simulink model "STFT_IP"  (R2021b)
settings: Solver=VariableStepAuto  StartTime=0.0  StopTime=2048*15/fs  RelTol=1e-3
InitFcn:
  | f = 12.288e6;
  | fs = 61.44e6;
  | N = 8;
  | n = 0:N-1;
  | Hamming = 0.54 - 0.46 * cos(2*pi*n/N);
  | Norm_Ham = sum(Hamming);
  | Hanning = 0.5 * (1 + cos(2*pi*n/N));
  | Norm_Han = sum(Hanning);
libraries: hdlBasic x52, hdlDSPIP x1, hdlsllib x1, vmcUtilities x1
settings Model: Creator=yxb20126  LastModifiedBy=yxb20126

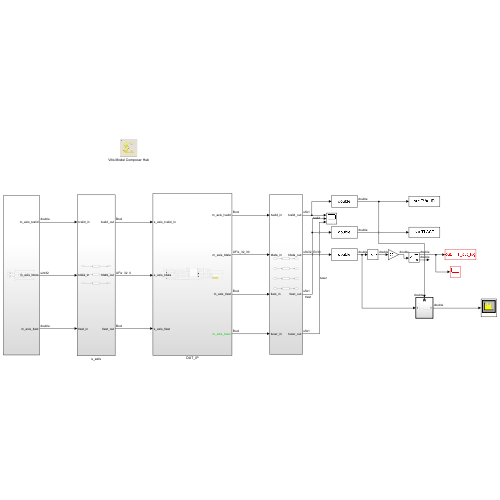
[thumbnail: Simulink's stored preview of the top-level diagram]
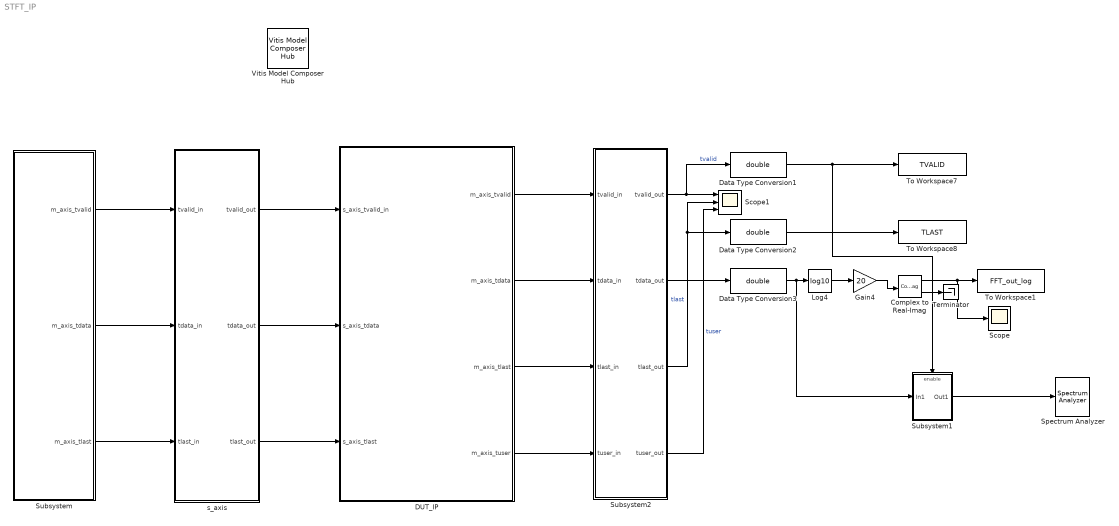
== system STFT_IP ==
  Complex to Real-Imag : ComplexToRealImag
  DUT_IP : Subsystem
  Data Type Conversion1 : DataTypeConversion  OutDataTypeStr=double  SaturateOnIntegerOverflow=on
  Data Type Conversion2 : DataTypeConversion  OutDataTypeStr=double  SaturateOnIntegerOverflow=on
  Data Type Conversion3 : DataTypeConversion  OutDataTypeStr=double  SaturateOnIntegerOverflow=on
  Gain4 : Gain  Gain=20
  Log4 : Math  Operator=log10  OutputSignalType=real  SaturateOnIntegerOverflow=on
  Scope : Scope
  Scope1 : Scope  NumInputPorts=3
  Spectrum Analyzer : SpectrumAnalyzer  IsFrequencyInputMode=1
  Subsystem : Subsystem
  Subsystem1 : Subsystem
  Subsystem2 : Subsystem
  Terminator : Terminator
  To Workspace1 : ToWorkspace  VariableName=FFT_out_log  SampleTime=-1
      settings: Save2DSignal=2-D array (concatenate along first dimension)
  To Workspace7 : ToWorkspace  VariableName=TVALID  SampleTime=1/fs
      settings: Save2DSignal=2-D array (concatenate along first dimension)
  To Workspace8 : ToWorkspace  VariableName=TLAST  SampleTime=1/fs
      settings: Save2DSignal=2-D array (concatenate along first dimension)
  Vitis Model Composer Hub : vmcUtilities/Vitis Model Composer Hub  Tag=genX  CodeGeneration=off  SubsystemName=<enter or select subsystem name>  TargetDirectory=./code  ExportType=HLS C++ code  IpVendor=xilinx.com  IpLibrary=hls  IpVersion=1.0  IpHWLanguage=Verilog  AieCompilerOptions={}  CreateTestbench=off  TestbenchStackSize=10  RunAieSim=off  AieSimTimeout=50000  RunAieSimProfiling=off  LaunchVitisAnalyzer=off  PlotOutput=off  RunX86Sim=off  X86SimTimeout=10  GenHwImage=off  PlatformType=Not Specified  HwSystemType=Baremetal  HwValidationTarget=hw  ProjDevice=xczu48dr-ffvg1517-2-e  ProjDevicePart=xczu48dr-ffvg1517-2-e  SamplePeriod=-1  ClockFrequency=200  DataPathParallelism=1  xilinxfamily=zynquplusRFSOC  part=xczu48dr  speed=-2-e  package=ffvg1517  directory=C:/Workspace/STFT  testbench=off  incr_netlist=off  synthesis_tool=Vivado  clock_wrapper=Clock Enables  dbl_ovrd=According to Block Masks  dcm_input_clock_period=10  sysclk_period=(1/fs)*10e9  simulink_period=1/fs  eval_field=0
  s_axis : Subsystem
  wires:
  Subsystem/1(m_axis_tvalid) -> s_axis/1(tvalid_in)
  Subsystem/2(m_axis_tdata) -> s_axis/2(tdata_in)
  Subsystem/3(m_axis_tlast) -> s_axis/3(tlast_in)
  s_axis/1(tvalid_out) -> DUT_IP/1(s_axis_tvalid_in)
  s_axis/2(tdata_out) -> DUT_IP/2(s_axis_tdata)
  s_axis/3(tlast_out) -> DUT_IP/3(s_axis_tlast)
  DUT_IP/4(m_axis_tuser) -> Subsystem2/4(tuser_in)
  Subsystem2/2(tdata_out) -> Data Type Conversion3/1
  Subsystem2/1(tvalid_out) -> Data Type Conversion1/1, Scope1/1  "tvalid"
  Subsystem2/3(tlast_out) -> Scope1/2, Data Type Conversion2/1  "tlast"
  Subsystem2/4(tuser_out) -> Scope1/3  "tuser"
  Data Type Conversion1/1 -> Subsystem1/Enable, To Workspace7/1
  Data Type Conversion2/1 -> To Workspace8/1
  Log4/1 -> Gain4/1
  Data Type Conversion3/1 -> Subsystem1/1(In1), Log4/1
  DUT_IP/1(m_axis_tvalid) -> Subsystem2/1(tvalid_in)
  DUT_IP/2(m_axis_tdata) -> Subsystem2/2(tdata_in)
  DUT_IP/3(m_axis_tlast) -> Subsystem2/3(tlast_in)
  Gain4/1 -> Complex to Real-Imag/1
  Complex to Real-Imag/1 -> Scope/1, To Workspace1/1
  Complex to Real-Imag/2 -> Terminator/1
  Subsystem1/1(Out1) -> Spectrum Analyzer/1

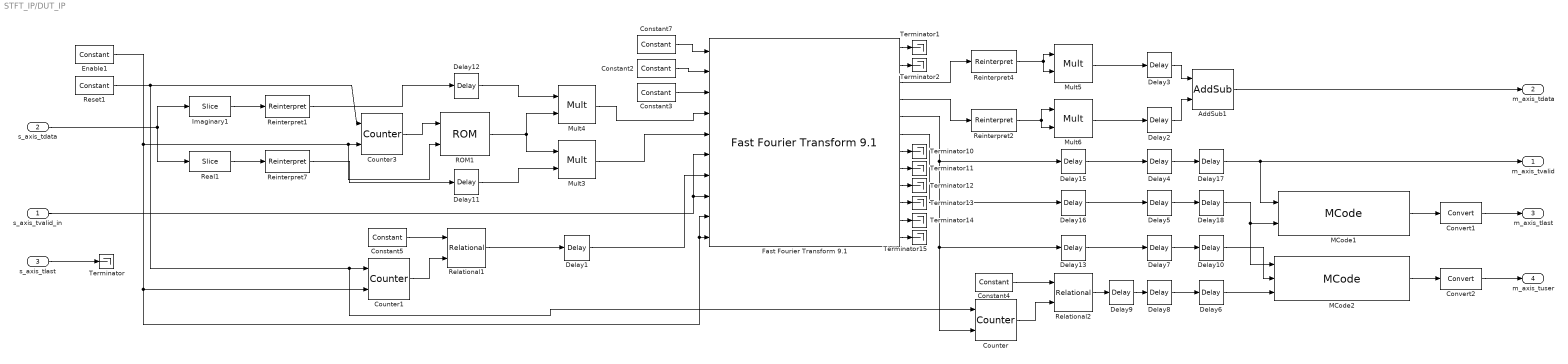
== system STFT_IP/DUT_IP ==
  s_axis_tvalid_in : Inport
  s_axis_tdata : Inport  Port=2
  s_axis_tlast : Inport  Port=3
  AddSub1 : hdlBasic/AddSub  mode=Addition  use_carryin=off  use_carryout=off  en=off  latency=1  precision=User Defined  arith_type=Unsigned  n_bits=32  bin_pt=30  quantization=Truncate  overflow=Saturate  use_behavioral_HDL=off  hw_selection=Fabric  pipelined=off  XmcBlockStatus=1  maskContainerNames=tabcontainer1  block_type=addsub  block_config=sysgen:Addsub_config
  Constant2 : hdlBasic/Constant  const=0  gui_display_data_type=Fixed-point  arith_type=Unsigned  n_bits=1  bin_pt=0  preci_type=Single  exp_width=8  frac_width=24  explicit_period=on  period=1/fs  XmcBlockStatus=1  maskContainerNames=tabcontainer1  block_type=constant  block_config=sysgen:Constant_config
  Constant3 : hdlBasic/Constant  const=0  gui_display_data_type=Boolean  arith_type=Boolean  n_bits=1  bin_pt=0  preci_type=Single  exp_width=8  frac_width=24  explicit_period=on  period=1/fs  XmcBlockStatus=1  maskContainerNames=tabcontainer1  block_type=constant  block_config=sysgen:Constant_config
  Constant4 : hdlBasic/Constant  const=N*1024-1  gui_display_data_type=Fixed-point  arith_type=Unsigned  n_bits=ceil(log2(N*1024))  bin_pt=0  preci_type=Single  exp_width=8  frac_width=24  explicit_period=on  period=1/fs  XmcBlockStatus=1  maskContainerNames=tabcontainer1  block_type=constant  block_config=sysgen:Constant_config
  Constant5 : hdlBasic/Constant  const=N-1  gui_display_data_type=Fixed-point  arith_type=Unsigned  n_bits=11  bin_pt=0  preci_type=Single  exp_width=8  frac_width=24  explicit_period=on  period=1/fs  XmcBlockStatus=1  maskContainerNames=tabcontainer1  block_type=constant  block_config=sysgen:Constant_config
  Constant7 : hdlBasic/Constant  const=0  gui_display_data_type=Fixed-point  arith_type=Unsigned  n_bits=12  bin_pt=0  preci_type=Single  exp_width=8  frac_width=24  explicit_period=on  period=1/fs  XmcBlockStatus=1  maskContainerNames=tabcontainer1  block_type=constant  block_config=sysgen:Constant_config
  Convert1 : hdlBasic/Convert  gui_display_data_type=Boolean  arith_type=Boolean  n_bits=16  bin_pt=14  float_type=Single  exp_bits=8  fraction_bits=24  quantization=Truncate  overflow=Wrap  en=off  latency=0  pipeline=off  XmcBlockStatus=1  maskContainerNames=group2  block_type=convert  block_config=sysgen:Convert_config
  Convert2 : hdlBasic/Convert  gui_display_data_type=Boolean  arith_type=Boolean  n_bits=16  bin_pt=14  float_type=Single  exp_bits=8  fraction_bits=24  quantization=Truncate  overflow=Wrap  en=off  latency=0  pipeline=off  XmcBlockStatus=1  maskContainerNames=group2  block_type=convert  block_config=sysgen:Convert_config
  Counter : hdlBasic/Counter  cnt_type=Count limited  cnt_to=N*1024-1  operation=Up  start_count=0  cnt_by_val=1  arith_type=Unsigned  n_bits=ceil(log2(N*1024))  bin_pt=0  load_pin=off  rst=on  en=on  explicit_period=Explicit  period=1/fs  use_behavioral_HDL=off  implementation=Fabric  XmcBlockStatus=1  maskContainerNames=group1  block_type=counter  block_config=sysgen:Counter_config
  Counter1 : hdlBasic/Counter  cnt_type=Count limited  cnt_to=N-1  operation=Up  start_count=0  cnt_by_val=1  arith_type=Unsigned  n_bits=11  bin_pt=0  load_pin=off  rst=on  en=on  explicit_period=Explicit  period=1/fs  use_behavioral_HDL=off  implementation=Fabric  XmcBlockStatus=1  maskContainerNames=group1  block_type=counter  block_config=sysgen:Counter_config
  Counter3 : hdlBasic/Counter  cnt_type=Count limited  cnt_to=N-1  operation=Up  start_count=0  cnt_by_val=1  arith_type=Unsigned  n_bits=ceil(log2(N))  bin_pt=0  load_pin=off  rst=on  en=on  explicit_period=Explicit  period=1/fs  use_behavioral_HDL=off  implementation=Fabric  XmcBlockStatus=1  maskContainerNames=group1  block_type=counter  block_config=sysgen:Counter_config
  Delay{1,13,15..16} (4 alike) : hdlBasic/Delay  rst=off  en=off  latency=3  reg_retiming=off  XmcBlockStatus=1  maskContainerNames=group1  block_type=delay  block_config=sysgen:Delay_config
  Delay{2..8,10..12,17..18} (12 alike) : hdlBasic/Delay  rst=off  en=off  latency=1  reg_retiming=off  XmcBlockStatus=1  maskContainerNames=group1  block_type=delay  block_config=sysgen:Delay_config
  Delay9 : hdlBasic/Delay  rst=off  en=off  latency=2  reg_retiming=off  XmcBlockStatus=1  maskContainerNames=group1  block_type=delay  block_config=sysgen:Delay_config
  Enable1 : hdlBasic/Constant  const=1  gui_display_data_type=Boolean  arith_type=Boolean  n_bits=11  bin_pt=0  preci_type=Single  exp_width=8  frac_width=24  explicit_period=on  period=1/fs  XmcBlockStatus=1  maskContainerNames=tabcontainer1  block_type=constant  block_config=sysgen:Constant_config
  Fast Fourier Transform 9.1 : hdlDSPIP/Fast Fourier Transform 9.1   transform_length=2048  target_clock_frequency=200  target_data_throughput=50  implementation_options=pipelined_streaming_io  run_time_configurable_transform_length=off  phase_factor_width=16  scaling_options=scaled  rounding_modes=truncation  aclken=on  aresetn=on  output_ordering=natural_order  cyclic_prefix_insertion=off  throttle_scheme=nonrealtime  xk_index=off  ovflo=off  trim_axipin_name=on  memory_options_data=block_ram  memory_options_phase_factors=block_ram  number_of_stages_using_block_ram_for_data_and_phase_factors=6  memory_options_reorder=block_ram  memory_options_hybrid=off  complex_mult_type=use_mults_resources  butterfly_type=use_luts  simulation_type=hybrid_sim  simulation_model=sysgen:xfftv9_cmodel  data_path_portlist={ 's_axis_data_tdata', 'm_axis_data_tdata', 'm_axis_status_tdata', 'event_fft_overflow' }  channels=1  input_ordering=natural_order  input_width=16  ip_name=Fast Fourier Transform  ip_version=9.1  dsptool_ready=true  ipcore_usecache=true  ipcore_useipmodelcache=true  wrapper_available=true  port_translation_map={ 'aclken' => 'en', 'aresetn' => 'rst'}  data_format=fixed_point  XmcBlockStatus=1  maskContainerNames=tabcontainer1  block_type=xfft_v9_1  block_config=sysgen:rodinimport_config
  Imaginary1 : hdlBasic/Slice  nbits=16  boolean_output=off  mode=Two Bit Locations  bit1=31  base1=LSB of Input  bit0=16  base0=LSB of Input  XmcBlockStatus=1  maskContainerNames=group1  block_type=slice  block_config=sysgen:Slice_config
  MCode1 : hdlBasic/MCode  mfname=EndOfFrame  explicit_period=on  period=1/fs  iptable={ 'FFT_TVALID', ''; 'FFT_TLAST', '' }  optable={ 'FrameEnd', 'off' }  enable_stdout=off  enable_debug=off  suppress_output='on'  defparams={}  hide_port_list={}  block_type=mcode
      settings: infoedit=Pass input values to a MATLAB function for evaluation in Xilinx fixed-point type. The input ports of the block are input arguments of the function. The output ports of the block are output arguments of the function.
  MCode2 : hdlBasic/MCode  mfname=StartOfFrame  explicit_period=on  period=1/fs  iptable={ 'FFT_TLAST', ''; 'FFT_TVALID', ''; 'FFT_END', '' }  optable={ 'FrameStart', 'off' }  enable_stdout=off  enable_debug=off  suppress_output='on'  defparams={}  hide_port_list={}  block_type=mcode
      settings: infoedit=Pass input values to a MATLAB function for evaluation in Xilinx fixed-point type. The input ports of the block are input arguments of the function. The output ports of the block are output arguments of the function.
  Mult3 : hdlBasic/Mult  precision=User Defined  arith_type="Signed  (2's comp)"  n_bits=16  bin_pt=15  quantization=Truncate  overflow=Saturate  en=off  latency=3  use_behavioral_HDL=off  opt=Speed  use_embedded=on  optimum_pipeline=off  pipeline=on  use_rpm=on  placement_style=Triangular  XmcBlockStatus=1  maskContainerNames=group1  block_type=mult  block_config=sysgen:Mult_config
  Mult4 : hdlBasic/Mult  precision=User Defined  arith_type="Signed  (2's comp)"  n_bits=16  bin_pt=15  quantization=Truncate  overflow=Saturate  en=off  latency=3  use_behavioral_HDL=off  opt=Speed  use_embedded=on  optimum_pipeline=off  pipeline=on  use_rpm=on  placement_style=Triangular  XmcBlockStatus=1  maskContainerNames=group1  block_type=mult  block_config=sysgen:Mult_config
  Mult5 : hdlBasic/Mult  precision=User Defined  arith_type=Unsigned  n_bits=32  bin_pt=31  quantization=Truncate  overflow=Saturate  en=off  latency=3  use_behavioral_HDL=off  opt=Speed  use_embedded=on  optimum_pipeline=off  pipeline=on  use_rpm=on  placement_style=Triangular  XmcBlockStatus=1  maskContainerNames=group1  block_type=mult  block_config=sysgen:Mult_config
  Mult6 : hdlBasic/Mult  precision=User Defined  arith_type=Unsigned  n_bits=32  bin_pt=31  quantization=Truncate  overflow=Saturate  en=off  latency=3  use_behavioral_HDL=off  opt=Speed  use_embedded=on  optimum_pipeline=off  pipeline=on  use_rpm=on  placement_style=Triangular  XmcBlockStatus=1  maskContainerNames=group1  block_type=mult  block_config=sysgen:Mult_config
  ROM1 : hdlBasic/ROM  depth=N  initVector=Hanning  distributed_mem=Block RAM  rst=off  init_reg=0  en=on  latency=1  gui_display_data_type=Fixed-point  arith_type=Unsigned  n_bits=16  bin_pt=15  preci_type=Single  exp_width=8  frac_width=24  optimize=Area  use_rpm=on  simulation_type=fast_sim  XmcBlockStatus=1  maskContainerNames=tabcontainer1  block_type=sprom  block_config=sysgen:SPROM_config
  Real1 : hdlBasic/Slice  nbits=16  boolean_output=off  mode=Two Bit Locations  bit1=15  base1=LSB of Input  bit0=0  base0=LSB of Input  XmcBlockStatus=1  maskContainerNames=group1  block_type=slice  block_config=sysgen:Slice_config
  Reinterpret1 : hdlBasic/Reinterpret  force_arith_type=on  arith_type="Signed  (2's comp)"  force_bin_pt=on  bin_pt=15  XmcBlockStatus=1  maskContainerNames=group1  block_type=reinterpret  block_config=sysgen:Reinterpret_config
  Reinterpret2 : hdlBasic/Reinterpret  force_arith_type=on  arith_type="Signed  (2's comp)"  force_bin_pt=off  bin_pt=31  XmcBlockStatus=1  maskContainerNames=group1  block_type=reinterpret  block_config=sysgen:Reinterpret_config
  Reinterpret4 : hdlBasic/Reinterpret  force_arith_type=on  arith_type="Signed  (2's comp)"  force_bin_pt=off  bin_pt=31  XmcBlockStatus=1  maskContainerNames=group1  block_type=reinterpret  block_config=sysgen:Reinterpret_config
  Reinterpret7 : hdlBasic/Reinterpret  force_arith_type=on  arith_type="Signed  (2's comp)"  force_bin_pt=on  bin_pt=15  XmcBlockStatus=1  maskContainerNames=group1  block_type=reinterpret  block_config=sysgen:Reinterpret_config
  Relational1 : hdlBasic/Relational  mode=a=b  op_type=Bool  en=off  latency=1  XmcBlockStatus=1  maskContainerNames=tabcontainer1  block_type=relational  block_config=sysgen:Relational_config
  Relational2 : hdlBasic/Relational  mode=a=b  op_type=Bool  en=off  latency=1  XmcBlockStatus=1  maskContainerNames=tabcontainer1  block_type=relational  block_config=sysgen:Relational_config
  Reset1 : hdlBasic/Constant  const=0  gui_display_data_type=Boolean  arith_type=Boolean  n_bits=11  bin_pt=0  preci_type=Single  exp_width=8  frac_width=24  explicit_period=on  period=1/fs  XmcBlockStatus=1  maskContainerNames=tabcontainer1  block_type=constant  block_config=sysgen:Constant_config
  Terminator{,1..2,10..15} (9 alike) : Terminator
  m_axis_tvalid : Outport
  m_axis_tdata : Outport  Port=2
  m_axis_tlast : Outport  Port=3
  m_axis_tuser : Outport  Port=4
  wires:
  s_axis_tlast/1 -> Terminator/1
  Imaginary1/1 -> Reinterpret1/1
  Fast Fourier Transform 9.1/5 -> Counter/2, Delay13/1, Delay15/1
  Delay12/1 -> Mult4/1
  Fast Fourier Transform 9.1/11 -> Terminator14/1
  Delay16/1 -> Delay5/1
  Constant3/1 -> Fast Fourier Transform 9.1/3
  Relational1/1 -> Delay1/1
  Delay1/1 -> Fast Fourier Transform 9.1/7
  Delay11/1 -> Mult3/2
  Counter1/1 -> Relational1/2
  Constant5/1 -> Relational1/1
  Fast Fourier Transform 9.1/2 -> Terminator2/1
  Fast Fourier Transform 9.1/1 -> Terminator1/1
  s_axis_tdata/1 -> Real1/1, Imaginary1/1
  Fast Fourier Transform 9.1/3 -> Reinterpret4/1
  Fast Fourier Transform 9.1/10 -> Terminator13/1
  Mult6/1 -> Delay2/1
  Fast Fourier Transform 9.1/7 -> Terminator10/1
  Mult4/1 -> Fast Fourier Transform 9.1/4
  Reinterpret4/1 -> Mult5/1, Mult5/2
  Reinterpret2/1 -> Mult6/1, Mult6/2
  Delay15/1 -> Delay4/1
  ROM1/1 -> Mult4/2, Mult3/1
  Fast Fourier Transform 9.1/8 -> Terminator11/1
  Fast Fourier Transform 9.1/12 -> Terminator15/1
  Counter3/1 -> ROM1/1
  Fast Fourier Transform 9.1/6 -> Delay16/1
  Constant2/1 -> Fast Fourier Transform 9.1/2
  Real1/1 -> Reinterpret7/1
  Fast Fourier Transform 9.1/9 -> Terminator12/1
  Fast Fourier Transform 9.1/4 -> Reinterpret2/1
  Mult5/1 -> Delay3/1
  s_axis_tvalid_in/1 -> Fast Fourier Transform 9.1/6, Fast Fourier Transform 9.1/8
  Reinterpret1/1 -> Delay12/1
  Enable1/1 -> Counter3/2, ROM1/2, Counter1/2, Fast Fourier Transform 9.1/10, Fast Fourier Transform 9.1/9
  Reinterpret7/1 -> Delay11/1
  Reset1/1 -> Counter/1, Counter1/1, Counter3/1
  MCode1/1 -> Convert1/1
  Mult3/1 -> Fast Fourier Transform 9.1/5
  Convert2/1 -> m_axis_tuser/1
  Convert1/1 -> m_axis_tlast/1
  AddSub1/1 -> m_axis_tdata/1
  Delay17/1 -> m_axis_tvalid/1, MCode1/1
  Constant4/1 -> Relational2/1
  Relational2/1 -> Delay9/1
  Delay18/1 -> MCode1/2, MCode2/1
  Delay6/1 -> MCode2/3
  Counter/1 -> Relational2/2
  Delay2/1 -> AddSub1/2
  Delay3/1 -> AddSub1/1
  Delay4/1 -> Delay17/1
  Delay5/1 -> Delay18/1
  Delay8/1 -> Delay6/1
  Constant7/1 -> Fast Fourier Transform 9.1/1
  Delay7/1 -> Delay10/1
  MCode2/1 -> Convert2/1
  Delay9/1 -> Delay8/1
  Delay10/1 -> MCode2/2
  Delay13/1 -> Delay7/1

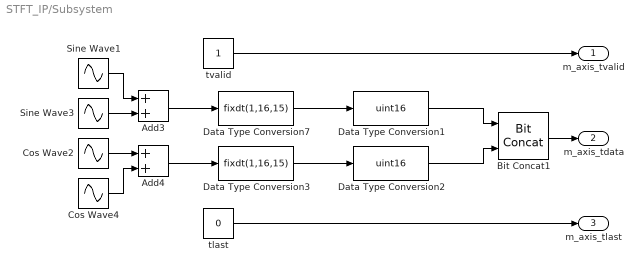
== system STFT_IP/Subsystem ==
  Add3 : Sum
  Add4 : Sum
  Bit Concat1 : hdlsllib/Logic and Bit Operations/Bit Concat  numInputs=2
  Cos Wave2 : Sin  Amplitude=0.4  Frequency=f*2*pi  Phase=pi/2  SampleTime=1/fs
  Cos Wave4 : Sin  Amplitude=0.4  Frequency=f*pi  Phase=pi/2  SampleTime=1/fs
  Data Type Conversion1 : DataTypeConversion  OutDataTypeStr=uint16  ConvertRealWorld=Stored Integer (SI)
  Data Type Conversion2 : DataTypeConversion  OutDataTypeStr=uint16  ConvertRealWorld=Stored Integer (SI)
  Data Type Conversion3 : DataTypeConversion  OutDataTypeStr=fixdt(1,16,15)  SaturateOnIntegerOverflow=on
  Data Type Conversion7 : DataTypeConversion  OutDataTypeStr=fixdt(1,16,15)  SaturateOnIntegerOverflow=on
  Sine Wave1 : Sin  Amplitude=0.4  Frequency=f*2*pi  SampleTime=1/fs
  Sine Wave3 : Sin  Amplitude=0.4  Frequency=f*pi  SampleTime=1/fs
  tlast : Constant  Value=0  SampleTime=1/fs
  tvalid : Constant  SampleTime=1/fs
  m_axis_tvalid : Outport
  m_axis_tdata : Outport  Port=2
  m_axis_tlast : Outport  Port=3
  wires:
  tlast/1 -> m_axis_tlast/1
  Data Type Conversion2/1 -> Bit Concat1/2
  Sine Wave1/1 -> Add3/1
  Cos Wave2/1 -> Add4/1
  Add3/1 -> Data Type Conversion7/1
  Sine Wave3/1 -> Add3/2
  Cos Wave4/1 -> Add4/2
  Data Type Conversion1/1 -> Bit Concat1/1
  Data Type Conversion3/1 -> Data Type Conversion2/1
  Add4/1 -> Data Type Conversion3/1
  Data Type Conversion7/1 -> Data Type Conversion1/1
  Bit Concat1/1 -> m_axis_tdata/1
  tvalid/1 -> m_axis_tvalid/1

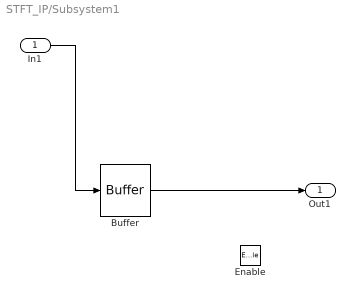
== system STFT_IP/Subsystem1 ==
  In1 : Inport
  Enable : EnablePort
  Buffer : Buffer  N=2048  OutputFrames=off
  Out1 : Outport
  wires:
  In1/1 -> Buffer/1
  Buffer/1 -> Out1/1

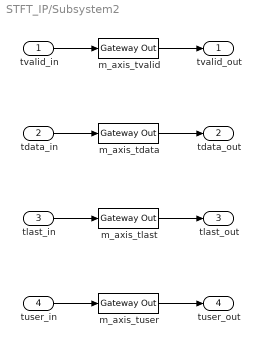
== system STFT_IP/Subsystem2 ==
  tvalid_in : Inport
  tdata_in : Inport  Port=2
  tlast_in : Inport  Port=3
  tuser_in : Inport  Port=4
  m_axis_tdata : hdlBasic/Gateway Out  inherit_from_input=on  hdl_port=on  rows=1  columns=1  UseAsDAC=off  DACChannel='1'  interface=None  automatic_assignment=on  address_offset=hex2dec('00')  intf_name=''  intf_description=''  timing_constraint=None  locs_specified=off  LOCs={}  io_standard={}  XmcBlockStatus=1  maskContainerNames=group4  block_type=gatewayout  block_config=sysgen:gateway_out_config  block_width_w=590  block_height_w=620  block_width=620  block_height=750
  m_axis_tlast : hdlBasic/Gateway Out  inherit_from_input=on  hdl_port=on  rows=1  columns=1  UseAsDAC=off  DACChannel='1'  interface=None  automatic_assignment=on  address_offset=hex2dec('00')  intf_name=''  intf_description=''  timing_constraint=None  locs_specified=off  LOCs={}  io_standard={}  XmcBlockStatus=1  maskContainerNames=group4  block_type=gatewayout  block_config=sysgen:gateway_out_config  block_width_w=590  block_height_w=620  block_width=620  block_height=750
  m_axis_tuser : hdlBasic/Gateway Out  inherit_from_input=on  hdl_port=on  rows=1  columns=1  UseAsDAC=off  DACChannel='1'  interface=None  automatic_assignment=on  address_offset=hex2dec('00')  intf_name=''  intf_description=''  timing_constraint=None  locs_specified=off  LOCs={}  io_standard={}  XmcBlockStatus=1  maskContainerNames=group4  block_type=gatewayout  block_config=sysgen:gateway_out_config  block_width_w=590  block_height_w=620  block_width=620  block_height=750
  m_axis_tvalid : hdlBasic/Gateway Out  inherit_from_input=on  hdl_port=on  rows=1  columns=1  UseAsDAC=off  DACChannel='1'  interface=None  automatic_assignment=on  address_offset=hex2dec('00')  intf_name=''  intf_description=''  timing_constraint=None  locs_specified=off  LOCs={}  io_standard={}  XmcBlockStatus=1  maskContainerNames=group4  block_type=gatewayout  block_config=sysgen:gateway_out_config  block_width_w=590  block_height_w=620  block_width=620  block_height=750
  tvalid_out : Outport
  tdata_out : Outport  Port=2
  tlast_out : Outport  Port=3
  tuser_out : Outport  Port=4
  wires:
  m_axis_tdata/1 -> tdata_out/1
  tlast_in/1 -> m_axis_tlast/1
  m_axis_tvalid/1 -> tvalid_out/1
  m_axis_tlast/1 -> tlast_out/1
  tvalid_in/1 -> m_axis_tvalid/1
  tdata_in/1 -> m_axis_tdata/1
  tuser_in/1 -> m_axis_tuser/1
  m_axis_tuser/1 -> tuser_out/1

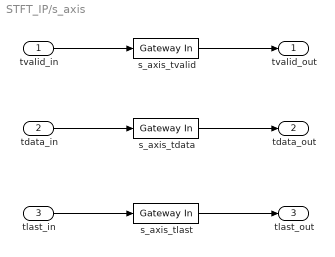
== system STFT_IP/s_axis ==
  tvalid_in : Inport
  tdata_in : Inport  Port=2
  tlast_in : Inport  Port=3
  s_axis_tdata : hdlBasic/Gateway In  gui_display_data_type=Fixed-point  arith_type=Unsigned  n_bits=32  bin_pt=0  preci_type=Single  exp_width=8  frac_width=24  rows=1  columns=1  quantization="Round  (unbiased: +/- Inf)"  overflow=Saturate  period=1/fs  UseAsADC=off  ADCChannel='1'  interface=None  automatic_assignment=on  address_offset=hex2dec('00')  intf_name=''  intf_description=''  default_value=0  timing_constraint=None  locs_specified=off  LOCs={}  io_standard={}  inherit_from_input=off  hdl_port=on  XmcBlockStatus=1  maskContainerNames=group4  block_type=gatewayin  block_config=sysgen:gateway_in_config  block_width_w=590  block_height_w=620  block_width=640  block_height=850
  s_axis_tlast : hdlBasic/Gateway In  gui_display_data_type=Boolean  arith_type=Boolean  n_bits=16  bin_pt=14  preci_type=Single  exp_width=8  frac_width=24  rows=1  columns=1  quantization="Round  (unbiased: +/- Inf)"  overflow=Saturate  period=1/fs  UseAsADC=off  ADCChannel='1'  interface=None  automatic_assignment=on  address_offset=hex2dec('00')  intf_name=''  intf_description=''  default_value=0  timing_constraint=None  locs_specified=off  LOCs={}  io_standard={}  inherit_from_input=off  hdl_port=on  XmcBlockStatus=1  maskContainerNames=group4  block_type=gatewayin  block_config=sysgen:gateway_in_config  block_width_w=590  block_height_w=620  block_width=640  block_height=850
  s_axis_tvalid : hdlBasic/Gateway In  gui_display_data_type=Boolean  arith_type=Boolean  n_bits=16  bin_pt=14  preci_type=Single  exp_width=8  frac_width=24  rows=1  columns=1  quantization="Round  (unbiased: +/- Inf)"  overflow=Saturate  period=1/fs  UseAsADC=off  ADCChannel='1'  interface=None  automatic_assignment=on  address_offset=hex2dec('00')  intf_name=''  intf_description=''  default_value=0  timing_constraint=None  locs_specified=off  LOCs={}  io_standard={}  inherit_from_input=off  hdl_port=on  XmcBlockStatus=1  maskContainerNames=group4  block_type=gatewayin  block_config=sysgen:gateway_in_config  block_width_w=590  block_height_w=620  block_width=640  block_height=850
  tvalid_out : Outport
  tdata_out : Outport  Port=2
  tlast_out : Outport  Port=3
  wires:
  s_axis_tdata/1 -> tdata_out/1
  s_axis_tlast/1 -> tlast_out/1
  s_axis_tvalid/1 -> tvalid_out/1
  tdata_in/1 -> s_axis_tdata/1
  tvalid_in/1 -> s_axis_tvalid/1
  tlast_in/1 -> s_axis_tlast/1
